simulink model "dc_motor_model"  (R2023a)
settings: Solver=VariableStepAuto  StartTime=0.0  StopTime=30.0  RelTol=1e-3
libraries: SignalEditorBlockLib x2, fuzblock x2, slpidlib x1
settings Model: Creator=Joe  LastModifiedBy=Joe

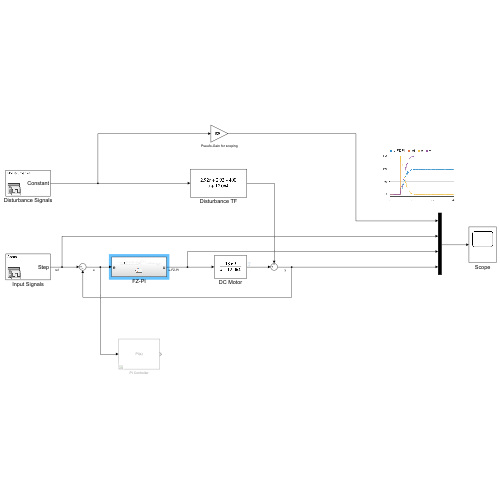
[thumbnail: Simulink's stored preview of the top-level diagram]
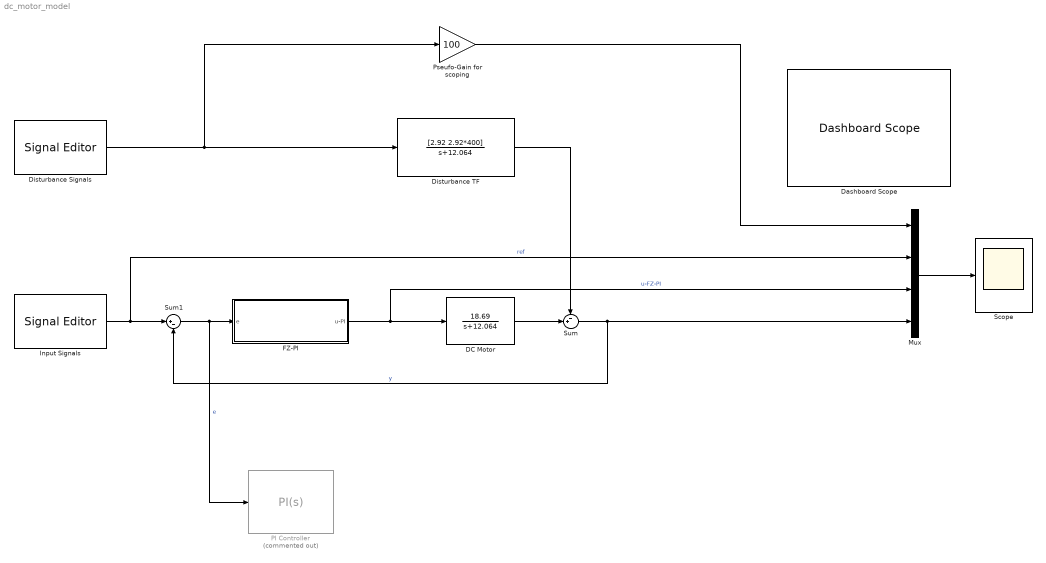
== system dc_motor_model ==
  DC Motor : TransferFcn  Numerator=[18.69]  Denominator=[1 12.064]
  Dashboard Scope : DashboardScope  TimeSpan=30  Ymin=0  Ymax=180
  Disturbance Signals : SignalEditorBlockLib/Signal Editor  FileName=external_disturbance.mat  ActiveScenario=NoDisturbance  ActiveSignal=Constant  IsBus=off  OutputBusObjectStr=Bus: BusObject  SampleTime=0  Interpolate=off  ZeroCross=off  OutputAfterFinalValue=Setting to zero  Unit=inherit  PreserveSignalName=on  ApplySigPropsToAllScenarios=on
  Disturbance TF : TransferFcn  Numerator=[2.92 2.92*400]  Denominator=[1 12.064]
  FZ-PI : Subsystem
  Input Signals : SignalEditorBlockLib/Signal Editor  FileName=input_scenarios.mat  ActiveScenario=Setup  ActiveSignal=Step  IsBus=off  OutputBusObjectStr=Bus: BusObject  SampleTime=0  Interpolate=off  ZeroCross=off  OutputAfterFinalValue=Setting to zero  Unit=V  PreserveSignalName=on  ApplySigPropsToAllScenarios=on
  Mux : Mux
  PI Controller : slpidlib/PID Controller  Commented=on  Controller=PI  Form=Parallel  TimeDomain=Continuous-time  UseExternalTs=off  SampleTime=-1  IntegratorMethod=Forward Euler  FilterMethod=Forward Euler  ControllerParametersSource=internal  P=0.918387293794384  I=12.6983083698527  UseKiTs=off  D=0  N=100  UseFilter=on  TunerSelectOption=Transfer Function Based (PID Tuner App)  InitialConditionSource=internal  InitialConditionForIntegrator=0  InitialConditionForFilter=0  DifferentiatorICPrevScaledInput=0  ExternalReset=none  TrackingMode=off  Kt=1  LimitOutput=off  SatLimitsSource=internal  UpperSaturationLimit=1  LowerSaturationLimit=-1  LinearizeAsGain=on  AntiWindupMode=clamping  Kb=1  LimitIntegrator=off  UpperIntegratorSaturationLimit=inf  LowerIntegratorSaturationLimit=-inf  RndMeth=Simplest  POutMin=[]  POutMax=[]  IOutMin=[]  IOutMax=[]  DOutMin=[]  DOutMax=[]  NOutMin=[]  NOutMax=[]  SumOutMin=[]  SumOutMax=[]  SaturationOutDataTypeStr=Inherit: Inherit via back propagation  SaturationOutMin=[]  SaturationOutMax=[]  PParamMin=[]  PParamMax=[]  IParamMin=[]  IParamMax=[]  DParamMin=[]  DParamMax=[]  NParamMin=[]  NParamMax=[]  KbParamMin=[]  KbParamMax=[]  KtParamMin=[]  KtParamMax=[]  KbOutMin=[]  KbOutMax=[]  KtOutMin=[]  KtOutMax=[]  IntegratorOutMin=[]  IntegratorOutMax=[]  FilterOutMin=[]  FilterOutMax=[]  SumI1OutMin=[]  SumI1OutMax=[]  SumI2OutMin=[]  SumI2OutMax=[]  SumI3OutMin=[]  SumI3OutMax=[]  SumI4OutMin=[]  SumI4OutMax=[]  SumDOutMin=[]  SumDOutMax=[]  DifferentiatorOutMin=[]  DifferentiatorOutMax=[]  FilterDiffOutCoefMin=[]  FilterDiffOutCoefMax=[]  ReciprocalOutMin=[]  ReciprocalOutMax=[]  SumDenOutMin=[]  SumDenOutMax=[]  SumNumOutMin=[]  SumNumOutMax=[]  DivideOutMin=[]  DivideOutMax=[]  UdiffTsProdOutMin=[]  UdiffTsProdOutMax=[]  NTsProdOutMin=[]  NTsProdOutMax=[]  UintegralTsProdOutMin=[]  UintegralTsProdOutMax=[]  UngainTsProdOutMin=[]  UngainTsProdOutMax=[]  ClampingZeroOutDataTypeStr=Inherit: Inherit via back propagation  ClampingZeroOutMin=[]  ClampingZeroOutMax=[]  FilterDenConstantOutDataTypeStr=Inherit: Inherit via back propagation  FilterDenConstantOutMin=[]  FilterDenConstantOutMax=[]  PCopyOutDataTypeStr=Inherit: Inherit via back propagation  PCopyOutMin=[]  PCopyOutMax=[]  NCopyOutDataTypeStr=Inherit: Inherit via back propagation  NCopyOutMin=[]  NCopyOutMax=[]  IntegratorContinuousStateAttributes=''  IntegratorStateMustResolveToSignalObject=off  IntegratorRTWStateStorageClass=Auto  FilterContinuousStateAttributes=''  FilterStateMustResolveToSignalObject=off  FilterRTWStateStorageClass=Auto  ParallelPVariant=InternalParameters  IdealPVariant=Disabled  IVariant=InternalParameters  DVariant=Disabled  IntegratorVariant=Continuous  SatVariant=Disabled  AWVariant=Passthrough  PCopyVariant=Disabled  TRVariant=Disabled  FdbkBlocksVariant=Forward  IdealPFdbkVariant=Disabled  SatFdbkVariant=Disabled  DerivativeFilterVariant=Disabled  NVariant=Disabled  NCopyVariant=Disabled_SignalSpec  FilterICVariant=Disabled  IntegratorICVariant=InternalICs  ExternalResetVariant=Disabled  TRSumVariant=Passthrough  SumFdbkVariant=Disabled  SumVariant=Sum_PI  TsampFilterVariant=InternalTs  TsampNgainVariant=Passthrough  TsampIntegralVariant=Disabled_SignalSpec  ExternalSaturationOutDataTypeStr=Inherit: Same as second input
      settings: LibrarySourceBlock=mcblib/Controls/Controllers/PI Controller
  Pseufo-Gain for scoping : Gain  Gain=100
  Scope : Scope
  Sum : Sum  Inputs=-+|
  Sum1 : Sum  Inputs=|+-
  wires:
  DC Motor/1 -> Sum/2
  Disturbance TF/1 -> Sum/1
  Disturbance Signals/1 -> Pseufo-Gain for scoping/1, Disturbance TF/1
  Sum/1 -> Sum1/2, Mux/4  "y"
  Pseufo-Gain for scoping/1 -> Mux/1
  Sum1/1 -> PI Controller/1, FZ-PI/1(e)  "e"
  Input Signals/1 -> Mux/2, Sum1/1  "ref"
  Mux/1 -> Scope/1
  FZ-PI/1(u-PI) -> Mux/3, DC Motor/1  "u-FZ-PI"

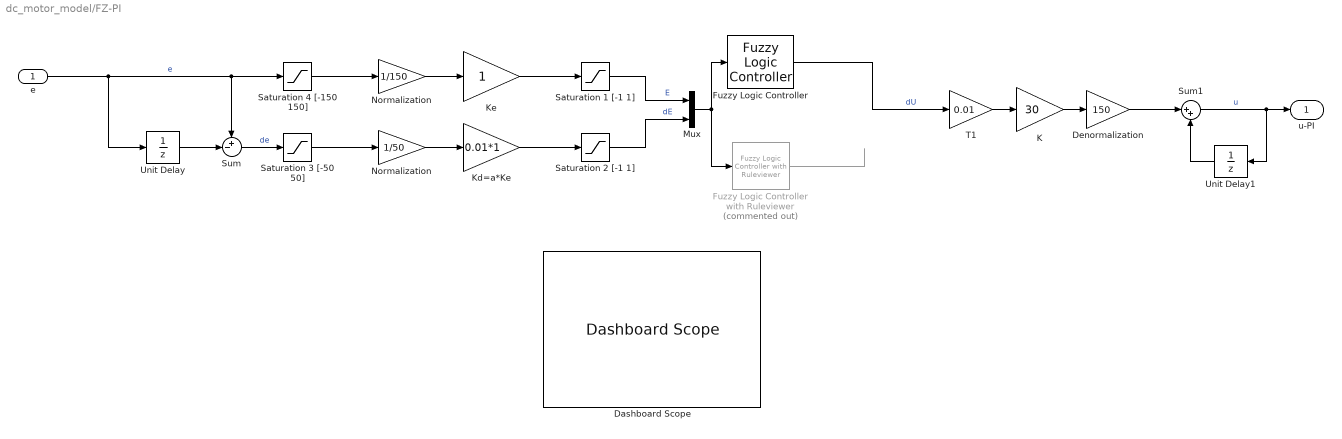
== system dc_motor_model/FZ-PI ==
  e : Inport
  Dashboard Scope : DashboardScope
  Denormalization : Gain  Gain=150
  Fuzzy Logic Controller : fuzblock/Fuzzy Logic  Controller  FIS=flc_fis  OutputSampleNumber=101  DataType=double  FuzzifiedInputs=off  RuleFiringStrengths=off  RuleOutputs=off  AggregatedOutputs=off  SimulateUsing=Interpreted execution  OutOfRangeInputValueMessage=warning  NoRuleFiredMessage=warning  EmptyOutputFuzzySetMessage=warning
  Fuzzy Logic Controller with Ruleviewer : fuzblock/Fuzzy Logic  Controller  with Ruleviewer  Commented=on  fismatrix=flc_fis  Ts=0.01
  K : Gain  Gain=30
  Kd=a*Ke : Gain  Gain=0.01*1
  Ke : Gain
  Mux : Mux  Inputs=2
  Normalization : Gain  Gain=1/50
  "Normalization " : Gain  Gain=1/150
  Saturation 1 [-1 1] : Saturate  UpperLimit=1  LowerLimit=-1
  Saturation 2 [-1 1] : Saturate  UpperLimit=1  LowerLimit=-1
  Saturation 3 [-50 50] : Saturate  UpperLimit=50  LowerLimit=-50
  Saturation 4 [-150 150] : Saturate  UpperLimit=150  LowerLimit=-150
  Sum : Sum  Inputs=+-|
  Sum1 : Sum  Inputs=|++
  T1 : Gain  Gain=0.01
  Unit Delay : UnitDelay  SampleTime=-1  HasFrameUpgradeWarning=on
  Unit Delay1 : UnitDelay  SampleTime=-1  HasFrameUpgradeWarning=on
  u-PI : Outport  VectorParamsAs1DForOutWhenUnconnected=off
  wires:
  Saturation 1 [-1 1]/1 -> Mux/1  "E"
  Unit Delay1/1 -> Sum1/2
  Denormalization/1 -> Sum1/1
  Unit Delay/1 -> Sum/2
  T1/1 -> K/1
  Saturation 2 [-1 1]/1 -> Mux/2  "dE"
  Ke/1 -> Saturation 1 [-1 1]/1
  Sum1/1 -> Unit Delay1/1, u-PI/1  "u"
  K/1 -> Denormalization/1
  Mux/1 -> Fuzzy Logic Controller with Ruleviewer/1, Fuzzy Logic Controller/1
  Sum/1 -> Saturation 3 [-50 50]/1  "de"
  e/1 -> Sum/1, Saturation 4 [-150 150]/1, Unit Delay/1  "e"
  Kd=a*Ke/1 -> Saturation 2 [-1 1]/1
  "Normalization "/1 -> Ke/1
  Saturation 3 [-50 50]/1 -> Normalization/1
  Normalization/1 -> Kd=a*Ke/1
  Saturation 4 [-150 150]/1 -> "Normalization "/1
  Fuzzy Logic Controller with Ruleviewer/1 -> ?
  Fuzzy Logic Controller/1 -> T1/1  "dU"
